simulink model "SFB_NL"  (Simulink 6.6)
settings: Solver=ode2  StartTime=0.0  StopTime=50  FixedStep=0.001  RelTol=1e-3
InitFcn:
  | linmod1
undefined symbols (not defined in the file or in its folder): a, dzcv, fc, fp, fs, g, j, K, l, M, mi, xc, yc
settings Model: Creator=AF1  LastModifiedBy=AF1
settings DataIOCC: SignalLoggingName=sigsOut
settings OptimizationCC: BooleanDataType=off
settings DebuggingCC: SignalResolutionControl=TryResolveAllWithWarning  SolverPrmCheckMsg=none  MultiTaskDSMMsg=warning  MultiTaskCondExecSysMsg=none  StrictBusMsg=None
settings HardwareCC: TargetUnknown=on
settings RTWCC: IncludeERTFirstTime=on

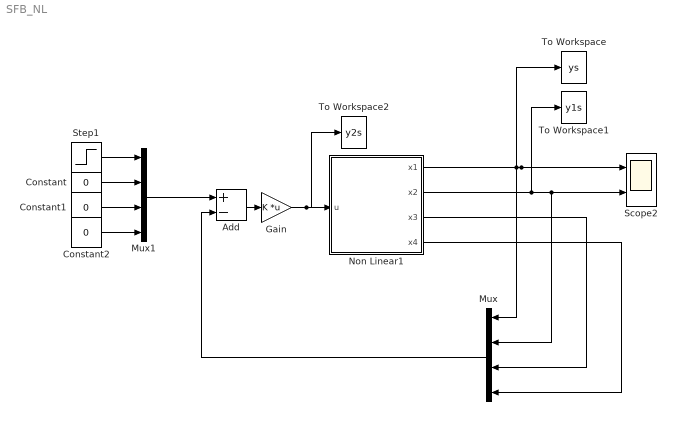
== system SFB_NL ==
  Add : Sum  Inputs=+-  OutScaling=2^-10
  Constant : Constant  Value=0
  Constant1 : Constant  Value=0
  Constant2 : Constant  Value=0
  Gain : Gain  Gain=K  Multiplication=Matrix(K*u)
  Mux : Mux  Orientation=left
  Mux1 : Mux
  Non Linear1 : Subsystem
  Scope2 : Scope  NumInputPorts=2
      settings: TimeRange=50  YMin=-0.05~-0.06  YMax=0.2~0.01000000000000001
  Step1 : Step  Time=20  After=0.2  SampleTime=0
  To Workspace : ToWorkspace  VariableName=ys  SampleTime=-1  SaveFormat=Structure With Time
  To Workspace1 : ToWorkspace  VariableName=y1s  SampleTime=-1  SaveFormat=Structure With Time
  To Workspace2 : ToWorkspace  VariableName=y2s  SampleTime=-1  SaveFormat=Structure With Time
  wires:
  Add/1 -> Gain/1
  Step1/1 -> Mux1/1
  Mux/1 -> Add/2
  Mux1/1 -> Add/1
  Constant/1 -> Mux1/2
  Constant1/1 -> Mux1/3
  Constant2/1 -> Mux1/4
  Gain/1 -> Non Linear1/1(u), To Workspace2/1
  Non Linear1/1(x1) -> Mux/1, Scope2/1, To Workspace/1
  Non Linear1/2(x2) -> Scope2/2, Mux/2, To Workspace1/1
  Non Linear1/3(x3) -> Mux/3
  Non Linear1/4(x4) -> Mux/4

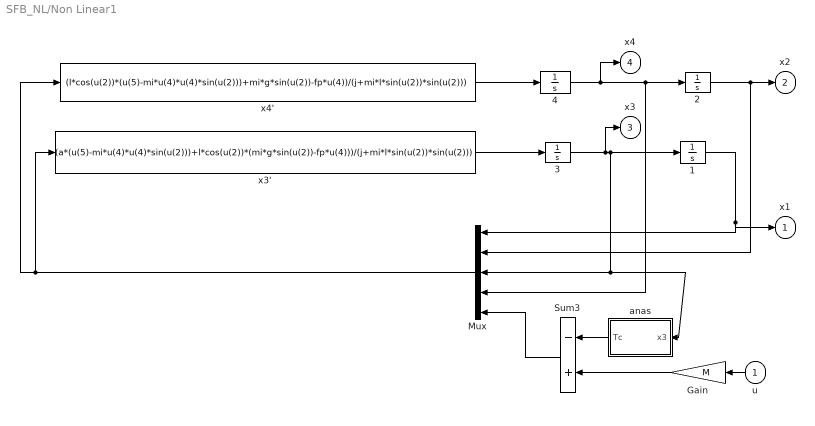
== system SFB_NL/Non Linear1 ==
  u : Inport  Orientation=left
  {1..4} (4 alike) : Integrator
  Gain : Gain  Orientation=left  Gain=M  SaturateOnIntegerOverflow=on
  Mux : Mux  Orientation=left  Inputs=5
  Sum3 : Sum  Orientation=left  Inputs=-+  SaturateOnIntegerOverflow=on
  anas : Subsystem  Orientation=left
  x3' : Fcn  Expr=(a*(u(5)-mi*u(4)*u(4)*sin(u(2)))+l*cos(u(2))*(mi*g*sin(u(2))-fp*u(4)))/(j+mi*l*sin(u(2))*sin(u(2)))
  x4' : Fcn  Expr=(l*cos(u(2))*(u(5)-mi*u(4)*u(4)*sin(u(2)))+mi*g*sin(u(2))-fp*u(4))/(j+mi*l*sin(u(2))*sin(u(2)))
  x1 : Outport
  x2 : Outport  Port=2
  x3 : Outport  Port=3
  x4 : Outport  Port=4
  wires:
  x3'/1 -> 3/1
  x4'/1 -> 4/1
  Sum3/1 -> Mux/5
  anas/1(Tc) -> Sum3/1
  Gain/1 -> Sum3/2
  2/1 -> x2/1, Mux/2
  3/1 -> x3/1, anas/1(x3), Mux/3, 1/1
  u/1 -> Gain/1
  Mux/1 -> x3'/1, x4'/1
  1/1 -> x1/1, Mux/1
  4/1 -> x4/1, Mux/4, 2/1

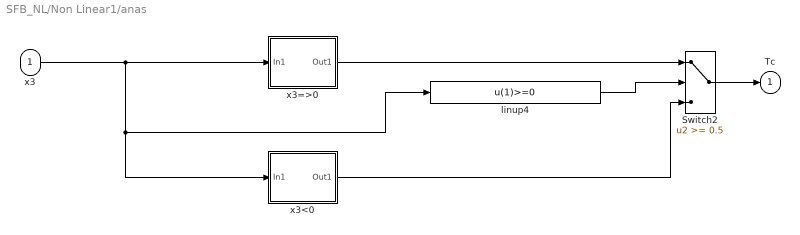
== system SFB_NL/Non Linear1/anas ==
  x3 : Inport
  Switch2 : Switch  Threshold=0.5  SaturateOnIntegerOverflow=on
  linup4 : Fcn  Expr=u(1)>=0
  x3<0 : Subsystem
  x3=>0 : Subsystem
  Tc : Outport  OutDataType=fixdt(1,16,0)  OutScaling=[]
  wires:
  linup4/1 -> Switch2/2
  Switch2/1 -> Tc/1
  x3<0/1(Out1) -> Switch2/3
  x3/1 -> linup4/1, x3<0/1(In1), x3=>0/1(In1)
  x3=>0/1(Out1) -> Switch2/1

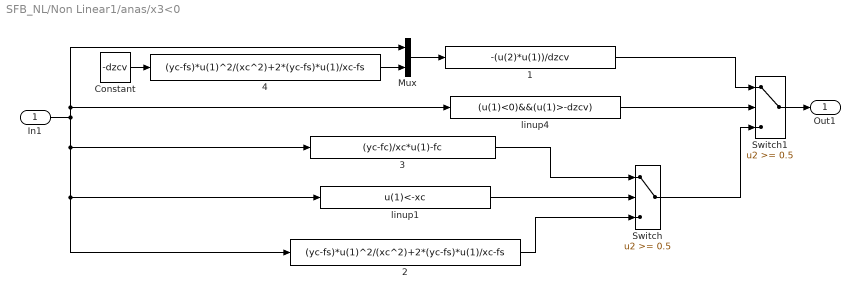
== system SFB_NL/Non Linear1/anas/x3<0 ==
  In1 : Inport
  1 : Fcn  Expr=-(u(2)*u(1))/dzcv
  2 : Fcn  Expr=(yc-fs)*u(1)^2/(xc^2)+2*(yc-fs)*u(1)/xc-fs
  3 : Fcn  Expr=(yc-fc)/xc*u(1)-fc
  4 : Fcn  Expr=(yc-fs)*u(1)^2/(xc^2)+2*(yc-fs)*u(1)/xc-fs
  Constant : Constant  Value=-dzcv
  Mux : Mux  Inputs=2
  Switch : Switch  Threshold=0.5  SaturateOnIntegerOverflow=on
  Switch1 : Switch  Threshold=0.5  SaturateOnIntegerOverflow=on
  linup1 : Fcn  Expr=u(1)<-xc
  linup4 : Fcn  Expr=(u(1)<0)&&(u(1)>-dzcv)
  Out1 : Outport
  wires:
  Constant/1 -> 4/1
  4/1 -> Mux/2
  Mux/1 -> 1/1
  3/1 -> Switch/1
  2/1 -> Switch/3
  1/1 -> Switch1/1
  linup4/1 -> Switch1/2
  linup1/1 -> Switch/2
  Switch/1 -> Switch1/3
  In1/1 -> Mux/1, linup4/1, 3/1, linup1/1, 2/1
  Switch1/1 -> Out1/1

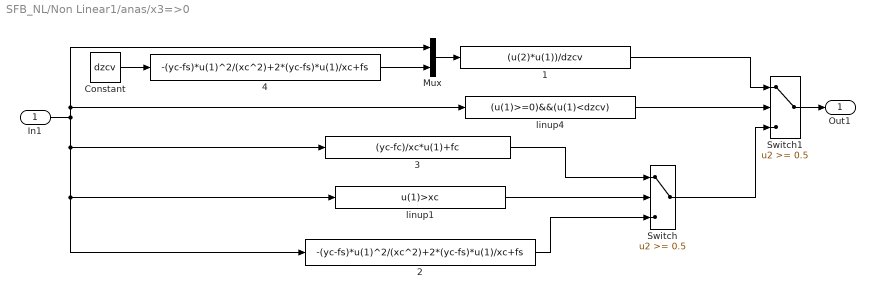
== system SFB_NL/Non Linear1/anas/x3=>0 ==
  In1 : Inport
  1 : Fcn  Expr=(u(2)*u(1))/dzcv
  2 : Fcn  Expr=-(yc-fs)*u(1)^2/(xc^2)+2*(yc-fs)*u(1)/xc+fs
  3 : Fcn  Expr=(yc-fc)/xc*u(1)+fc
  4 : Fcn  Expr=-(yc-fs)*u(1)^2/(xc^2)+2*(yc-fs)*u(1)/xc+fs
  Constant : Constant  Value=dzcv
  Mux : Mux  Inputs=2
  Switch : Switch  Threshold=0.5  SaturateOnIntegerOverflow=on
  Switch1 : Switch  Threshold=0.5  SaturateOnIntegerOverflow=on
  linup1 : Fcn  Expr=u(1)>xc
  linup4 : Fcn  Expr=(u(1)>=0)&&(u(1)<dzcv)
  Out1 : Outport
  wires:
  Constant/1 -> 4/1
  4/1 -> Mux/2
  Mux/1 -> 1/1
  Switch1/1 -> Out1/1
  In1/1 -> Mux/1, linup4/1, 2/1, linup1/1, 3/1
  Switch/1 -> Switch1/3
  linup1/1 -> Switch/2
  linup4/1 -> Switch1/2
  1/1 -> Switch1/1
  2/1 -> Switch/3
  3/1 -> Switch/1
